simulink library "sm_boom_lift_crawler_sensors"  (R2026a)
settings: Solver=VariableStepAuto
libraries: simulink x6
Description:
  | Boom Lift Crawler Sensors (Library)
  | 
  | Copyright 2020-2026 The MathWorks, Inc.
settings Model: Creator=smiller  LastModifiedBy=smiller

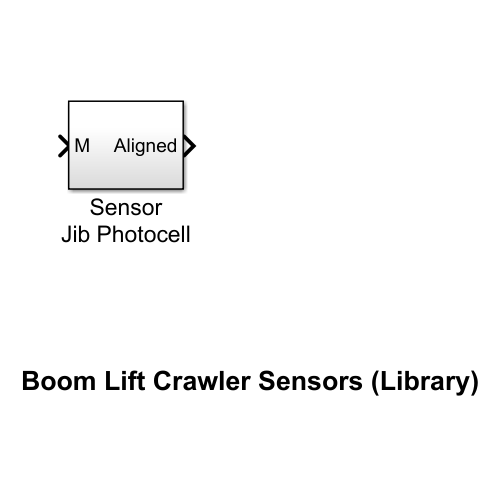
[thumbnail: Simulink's stored preview of the top-level diagram]
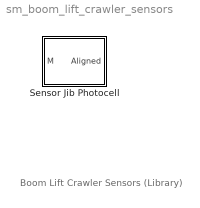
== system sm_boom_lift_crawler_sensors ==
  note: Boom Lift Crawler Sensors (Library)
  Sensor Jib Photocell : Subsystem

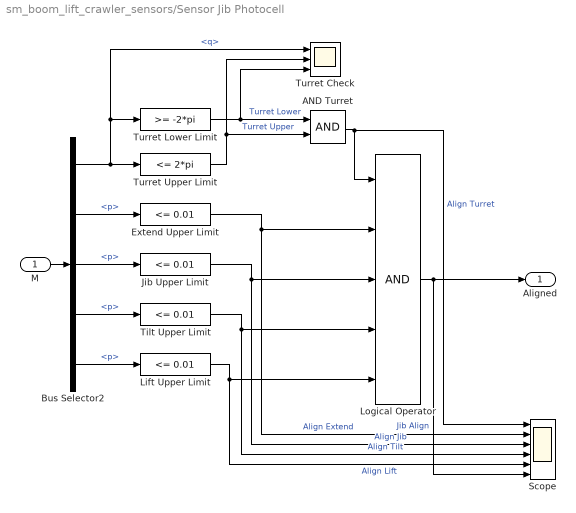
== system sm_boom_lift_crawler_sensors/Sensor Jib Photocell ==
  M : Inport
  AND Turret : Logic  AllPortsSameDT=off  OutDataTypeStr=boolean
  Bus Selector2 : BusSelector  OutputSignals=Mech.Turret.q,Mech.Extend.p,Mech.Jib.p,Mech.Tilt.p,Mech.Lift.p
  Extend Upper Limit : simulink/Logic and Bit Operations/Compare To Constant  relop=<=  const=0.01  OutDataTypeStr=boolean  ZeroCross=off
  Jib Upper Limit : simulink/Logic and Bit Operations/Compare To Constant  relop=<=  const=0.01  OutDataTypeStr=boolean  ZeroCross=off
  Lift Upper Limit : simulink/Logic and Bit Operations/Compare To Constant  relop=<=  const=0.01  OutDataTypeStr=boolean  ZeroCross=off
  Logical Operator : Logic  Inputs=5  AllPortsSameDT=off  OutDataTypeStr=boolean
  Scope : Scope  NumInputPorts=6
      settings: ActiveDisplayYMinimum=-0.125  ActiveDisplayYMaximum=1.125
  Tilt Upper Limit : simulink/Logic and Bit Operations/Compare To Constant  relop=<=  const=0.01  OutDataTypeStr=boolean  ZeroCross=off
  Turret Check : Scope  NumInputPorts=3
      settings: ActiveDisplayYMinimum=-1.29301  ActiveDisplayYMaximum=11.63709  DataLoggingVariableName=ScopeData2
  Turret Lower Limit : simulink/Logic and Bit Operations/Compare To Constant  relop=>=  const=-2*pi  OutDataTypeStr=boolean  ZeroCross=off
  Turret Upper Limit : simulink/Logic and Bit Operations/Compare To Constant  relop=<=  const=2*pi  OutDataTypeStr=boolean  ZeroCross=off
  Aligned : Outport
  wires:
  Logical Operator/1 -> Aligned/1, Scope/6  "Jib Align"
  Bus Selector2/1 -> Turret Upper Limit/1, Turret Check/1, Turret Lower Limit/1  "<q>"
  M/1 -> Bus Selector2/1
  Bus Selector2/5 -> Lift Upper Limit/1  "<p>"
  Bus Selector2/4 -> Tilt Upper Limit/1  "<p>"
  Bus Selector2/3 -> Jib Upper Limit/1  "<p>"
  Bus Selector2/2 -> Extend Upper Limit/1  "<p>"
  Turret Lower Limit/1 -> Turret Check/3, AND Turret/1  "Turret Lower"
  Turret Upper Limit/1 -> Turret Check/2, AND Turret/2  "Turret Upper"
  Extend Upper Limit/1 -> Scope/2, Logical Operator/2  "Align Extend"
  Jib Upper Limit/1 -> Scope/3, Logical Operator/3  "Align Jib"
  Tilt Upper Limit/1 -> Scope/4, Logical Operator/4  "Align Tilt"
  Lift Upper Limit/1 -> Scope/5, Logical Operator/5  "Align Lift"
  AND Turret/1 -> Logical Operator/1, Scope/1  "Align Turret"
